simulink model "demowf3"  (Simulink 6.1)
settings: Solver=ode4  StartTime=0.0  StopTime=200  FixedStep=0.1  RelTol=1e-3
libraries: simulink_extras x5, marine_gnc x5, simulink x2
settings Model: LastModifiedBy=Smogeli
settings DataIOCC: SignalLoggingName=sigsOut
settings OptimizationCC: BooleanDataType=off
settings HardwareCC: TargetUnknown=on
settings GRTTargetCC: ModelReferenceCompliant=off  MatFileLogging=off

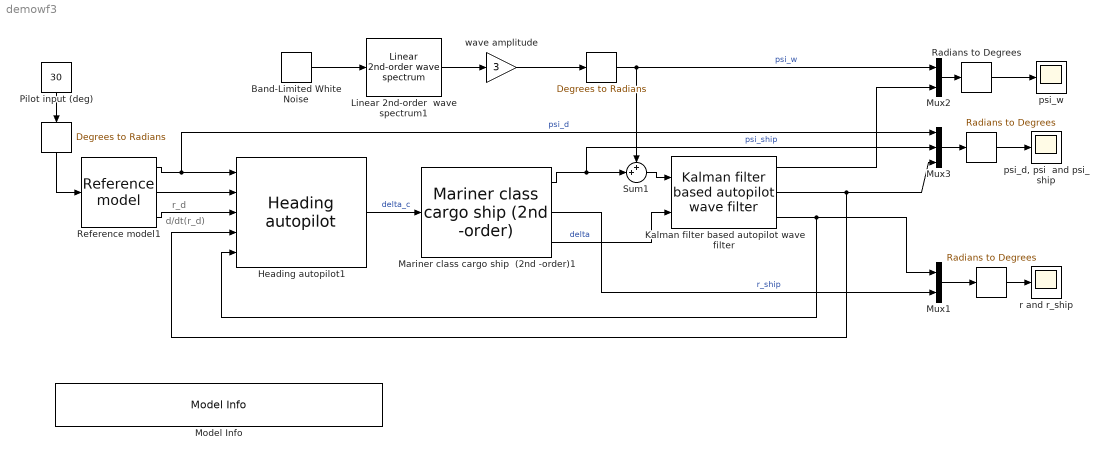
== system demowf3 ==
  note: r_d
  note: d/dt(r_d)
  " " : simulink_extras/Transformations/Radians to Degrees
  "  " : simulink_extras/Transformations/Radians to Degrees
  "   " : simulink_extras/Transformations/Degrees to Radians
  "     " : simulink_extras/Transformations/Degrees to Radians  Orientation=down
  Band-Limited White Noise : simulink/Sources/Band-Limited White Noise  Cov=[1]  Ts=0.1  seed=[23341]
  Heading autopilot1 : marine_gnc/Control/Autopilots/Heading autopilot  T_nomoto=107.3  K_nomoto=0.185  Kp=2  Td=50  Ti=100
  Kalman filter based autopilot wave filter : marine_gnc/Navigation/Observers/Kalman filter based autopilot wave filter  lambda=0.1  w_o=1.2  T_b=1000  K=0.185  T=107.3  r=1  q1=100  q2=0.01  q3=0.01  P0=1*eye(5)
  Linear 2nd-order  wave spectrum1 : marine_gnc/Environment/Waves/Linear 2nd-order  wave spectrum  sigma=.5  w_0=1.2  lambda=0.1
  Mariner class cargo ship  (2nd -order)1 : marine_gnc/Examples/Vessels/Mariner class cargo ship  (2nd -order)  rate_max=5*(pi/180)  delta_max=20*(pi/180)  K=0.185  T1=118  T2=7.8  T3=18.5
  Model Info : simulink/Model-Wide Utilities/Model Info  InitialBlockCM=None  BlockCM=None  Frame=on  DisplayStringWithTags=|  HorizontalTextAlignment=Left  LeftAlignmentValue=0.02  SourceBlockDiagram=demowf3  TagMaxNumber=20
      | Kalman filter based wave filter demo using compass measurements
      | %<Creator>Author: Thor I. Fossen
      | %<LastModificationDate>
  Mux1 : Mux  Inputs=2
  Mux2 : Mux  Inputs=2
  Mux3 : Mux  Inputs=3
  Pilot input (deg) : Constant  Orientation=down  Value=30
  "Radians to Degrees  " : simulink_extras/Transformations/Radians to Degrees
  Reference model1 : marine_gnc/Guidance/Reference model  v_max=1.0  zeta_d=1.0  w_d=0.1
  Sum1 : Sum  Inputs=++|  SaturateOnIntegerOverflow=on  InputSameDT=on
  "psi_d, psi  and psi_ship" : Scope
      settings: TimeRange=200  YMin=0  YMax=35  SaveName=ScopeData2  Decimation=10
  psi_w : Scope
      settings: TimeRange=200  YMin=-1.5  YMax=1.5  Decimation=10
  r and r_ship : Scope
      settings: TimeRange=200  YMin=-0.1  YMax=0.9  SaveName=ScopeData3  Decimation=10
  wave amplitude : Gain  Gain=3  SaturateOnIntegerOverflow=on
  wires:
  Band-Limited White Noise/1 -> Linear 2nd-order  wave spectrum1/1
  Mux2/1 -> "Radians to Degrees  "/1
  "Radians to Degrees  "/1 -> psi_w/1
  " "/1 -> "psi_d, psi  and psi_ship"/1
  Mux1/1 -> "  "/1
  "  "/1 -> r and r_ship/1
  Linear 2nd-order  wave spectrum1/1 -> wave amplitude/1
  Mux3/1 -> " "/1
  Mariner class cargo ship  (2nd -order)1/3 -> Kalman filter based autopilot wave filter/2  "delta"
  wave amplitude/1 -> "   "/1
  Heading autopilot1/1 -> Mariner class cargo ship  (2nd -order)1/1  "delta_c"
  Kalman filter based autopilot wave filter/2 -> Mux3/3, Heading autopilot1/4
  Kalman filter based autopilot wave filter/3 -> Mux1/1, Heading autopilot1/5
  Mariner class cargo ship  (2nd -order)1/1 -> Sum1/2, Mux3/2  "psi_ship"
  Sum1/1 -> Kalman filter based autopilot wave filter/1
  "   "/1 -> Sum1/1, Mux2/1  "psi_w"
  Mariner class cargo ship  (2nd -order)1/2 -> Mux1/2  "r_ship"
  Reference model1/1 -> Mux3/1, Heading autopilot1/1  "psi_d"
  Reference model1/2 -> Heading autopilot1/2
  Reference model1/3 -> Heading autopilot1/3
  Kalman filter based autopilot wave filter/1 -> Mux2/2
  Pilot input (deg)/1 -> "     "/1
  "     "/1 -> Reference model1/1
